simulink model "PVcelija"  (R2018a)
settings: Solver=VariableStepAuto  StartTime=0.0  StopTime=1  RelTol=1e-3
values from neighbouring files (symbols this model uses):
  G = 0.001    [PVcell.m]
  Gc = [1000 1000 1000 1000 400]    [BypassDiode.m]    (also in PVcell.m = 400; UIModulaG.m = i*200; UIModulaT.m = 1000; Untitled6.m = [Gc1 Gc1 Gc2 Gc2])
  k = k+1    (= 2)    [DailyInsolation.m]    (also in PVcell.m = 1.38e-23)
  q = 1.602e-19    [PVcell.m]
  Rp = 6.6    [PVcell.m]
  Rs = 0.005    [PVcell.m]
libraries: simulink x2
settings Model: Creator=User  LastModifiedBy=User

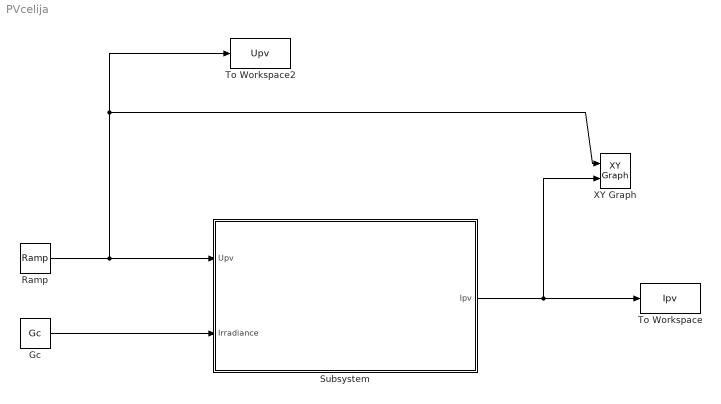
== system PVcelija ==
  Gc : Constant  Value=Gc
  Ramp : simulink/Sources/Ramp  slope=0.7  start=0  InitialOutput=0
  Subsystem : Subsystem
  To Workspace : ToWorkspace  VariableName=Ipv  SampleTime=-1
  To Workspace2 : ToWorkspace  VariableName=Upv  SampleTime=-1
  XY Graph : simulink/Sinks/XY Graph  xmin=0  xmax=0.6  ymin=0  ymax=1.2  st=-1
  wires:
  Subsystem/1(Ipv) -> XY Graph/2, To Workspace/1
  Gc/1 -> Subsystem/2(Irradiance)
  Ramp/1 -> To Workspace2/1, XY Graph/1, Subsystem/1(Upv)

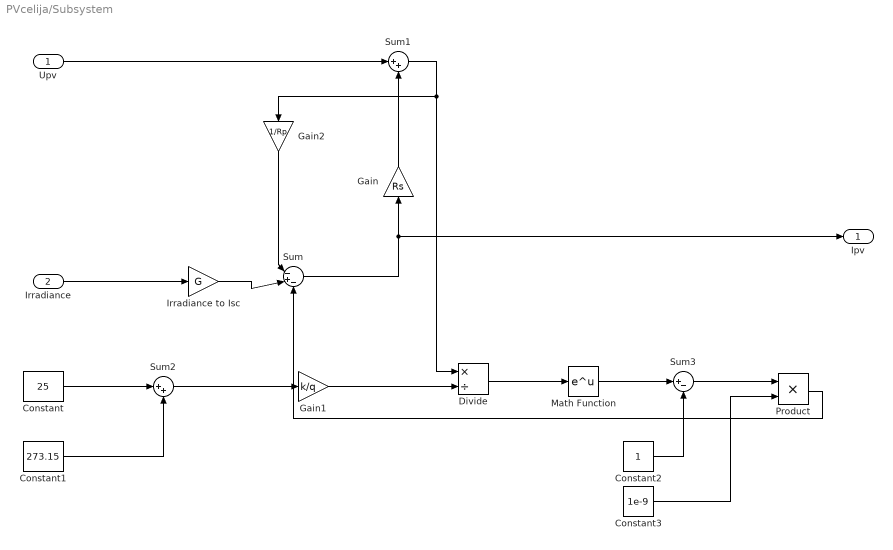
== system PVcelija/Subsystem ==
  Upv : Inport
  Irradiance : Inport  Port=2
  Constant : Constant  Value=25
  Constant1 : Constant  Value=273.15
  Constant2 : Constant
  Constant3 : Constant  Value=1e-9
  Divide : Product  Inputs=*/
  Gain : Gain  Gain=Rs
  Gain1 : Gain  Gain=k/q
  Gain2 : Gain  Gain=1/Rp
  "Irradiance to Isc " : Gain  Gain=G
  Math Function : Math  SaturateOnIntegerOverflow=on
  Product : Product
  Sum : Sum  Inputs=|-+-
  Sum1 : Sum  Inputs=|++
  Sum2 : Sum  Inputs=|++
  Sum3 : Sum  Inputs=|+-
  Ipv : Outport
  wires:
  Irradiance/1 -> "Irradiance to Isc "/1
  "Irradiance to Isc "/1 -> Sum/2
  Upv/1 -> Sum1/1
  Sum/1 -> Ipv/1, Gain/1
  Gain/1 -> Sum1/2
  Constant/1 -> Sum2/1
  Constant1/1 -> Sum2/2
  Sum2/1 -> Gain1/1
  Gain1/1 -> Divide/2
  Sum1/1 -> Gain2/1, Divide/1
  Gain2/1 -> Sum/1
  Divide/1 -> Math Function/1
  Math Function/1 -> Sum3/1
  Constant2/1 -> Sum3/2
  Sum3/1 -> Product/1
  Constant3/1 -> Product/2
  Product/1 -> Sum/3
